simulink model "simulation_rejection_periodic"  (Simulink 6.3)
settings: Solver=ode45  StartTime=0.0  StopTime=5000  RelTol=1e-3
libraries: cstblocks x4, simulink x1
settings Model: Creator=fromion  LastModifiedBy=xavier.litrico  ExtModeTrigMode=oneshot  ExtModeArmWhenConnect=off  ExtModeAutoUpdateStatusClock=off  BufferReuse=off
settings DataIOCC: InitialState=[]  LimitDataPoints=off  LoadInitialState=on
settings OptimizationCC: BlockReduction=off  BooleanDataType=off  InlineParams=on  BufferReuse=off
settings DebuggingCC: SolverPrmCheckMsg=none
settings HardwareCC: TargetUnknown=on

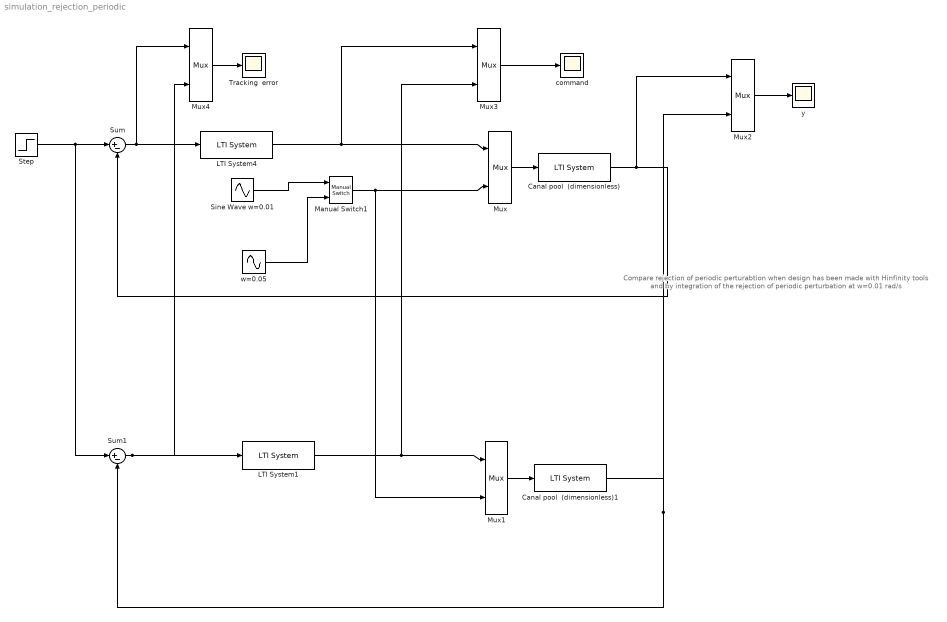
== system simulation_rejection_periodic ==
  note: Compare  rejection of periodic perturabtion
      | when design has been made with Hinfinity tools
      | and by integration of  the rejection  of periodic
      | perturbation at w=0.01 rad/s
  Canal pool  (dimensionless) : cstblocks/LTI System  sys=sys_bo_ss  IC=0
  Canal pool  (dimensionless)1 : cstblocks/LTI System  sys=sys_bo_ss  IC=0
  LTI System1 : cstblocks/LTI System  sys=K_PI_ss  IC=0
  LTI System4 : cstblocks/LTI System  sys=K_hinf_ss  IC=0
  Manual Switch1 : simulink/Signal Routing/Manual Switch  sw=1  action=0
  Mux{,1..4} (5 alike) : Mux  Inputs=2
  Sine Wave w=0.01 : Sin  Frequency=0.01  SampleTime=0
  Step : Step  SampleTime=0
  Sum : Sum  Inputs=|+-  SaturateOnIntegerOverflow=on  InputSameDT=on
  Sum1 : Sum  Inputs=|+-  SaturateOnIntegerOverflow=on  InputSameDT=on
  Tracking  error : Scope
      settings: SaveName=e  DataFormat=Array
  command : Scope
      settings: SaveName=u  DataFormat=Array
  w=0.05 : Sin  Frequency=0.05  SampleTime=0
  y : Scope
      settings: TimeRange=10000  YMin=-0.1  YMax=1.3  SaveName=y  DataFormat=Array  SampleTime=0.1
  wires:
  Sum/1 -> LTI System4/1, Mux4/1
  Canal pool  (dimensionless)/1 -> Sum/2, Mux2/1
  LTI System4/1 -> Mux/1, Mux3/1
  Mux/1 -> Canal pool  (dimensionless)/1
  Manual Switch1/1 -> Mux/2, Mux1/2
  Sum1/1 -> LTI System1/1, Mux4/2
  Canal pool  (dimensionless)1/1 -> Sum1/2, Mux2/2
  LTI System1/1 -> Mux1/1, Mux3/2
  Mux1/1 -> Canal pool  (dimensionless)1/1
  Mux2/1 -> y/1
  Mux3/1 -> command/1
  Mux4/1 -> Tracking  error/1
  Step/1 -> Sum/1, Sum1/1
  Sine Wave w=0.01/1 -> Manual Switch1/1
  w=0.05/1 -> Manual Switch1/2
